simulink model "CntroInput"  (R2016b)
settings: Solver=FixedStepAuto  StartTime=0.0  StopTime=10.0  RelTol=1e-3  SampleTimeConstraint=STIndependent
undefined symbols (not defined in the file): MPCSampleTime
libraries: simulink x7
settings Model: Creator=UAVLAB  LastModifiedBy=UAVLAB

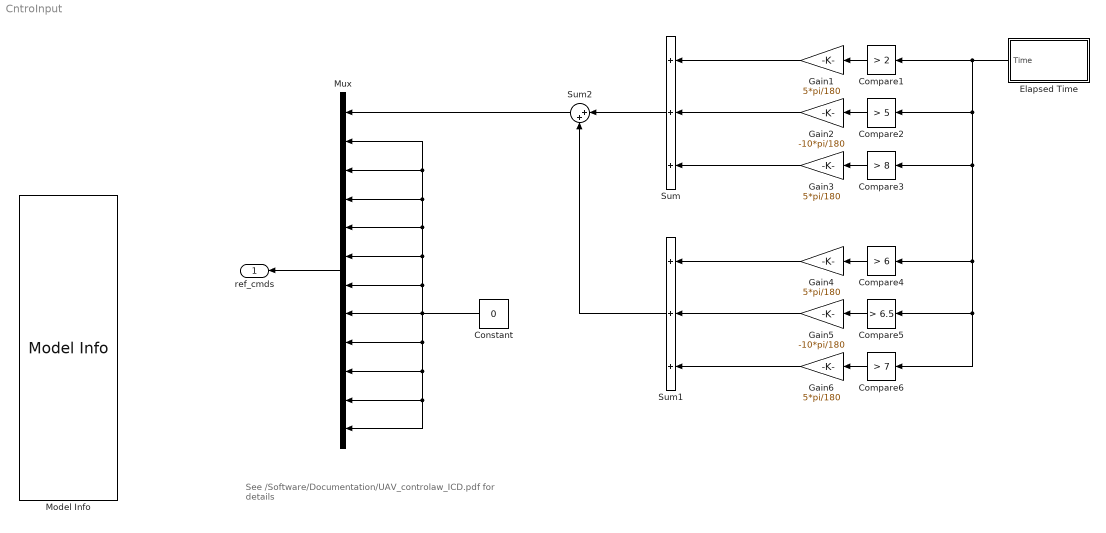
== system CntroInput ==
  note: See /Software/Documentation/UAV_controlaw_ICD.pdf
      | for details
  Compare1 : simulink/Logic and Bit Operations/Compare To Constant  relop=>  const=2  OutDataTypeStr=boolean
  Compare2 : simulink/Logic and Bit Operations/Compare To Constant  relop=>  const=5  OutDataTypeStr=boolean
  Compare3 : simulink/Logic and Bit Operations/Compare To Constant  relop=>  const=8  OutDataTypeStr=boolean
  Compare4 : simulink/Logic and Bit Operations/Compare To Constant  relop=>  const=6  OutDataTypeStr=boolean
  Compare5 : simulink/Logic and Bit Operations/Compare To Constant  relop=>  const=6.5  OutDataTypeStr=boolean
  Compare6 : simulink/Logic and Bit Operations/Compare To Constant  relop=>  const=7  OutDataTypeStr=boolean
  Constant : Constant  Value=0  SampleTime=-1
  Elapsed Time : Subsystem
  Gain{1,3..4,6} (4 alike) : Gain  Gain=5*pi/180  OutDataTypeStr=double
  Gain2 : Gain  Gain=-10*pi/180  OutDataTypeStr=double
  Gain5 : Gain  Gain=-10*pi/180  OutDataTypeStr=double
  Model Info : simulink/Model-Wide Utilities/Model Info  Frame=on  DisplayStringWithTags=|  HorizontalTextAlignment=Center  LeftAlignmentValue=0.5  SourceBlockDiagram=control_input2  TagMaxNumber=20
      | Ref Cmd Port Info
      | 
      | 1. phi_cmd
      | 2. theta_cmd
      | 3. psi_cmd
      | 4. p_cmd
      | 5. q_cmd
      | 6. r_cmd
      | 7. V_s_cmd
      | 8. h_cmd
      | 9. gndtrk_cmd
      | 10. aoa_cmd
      | 11. aos_cmd
      | 12. gamma_cmd
  Mux : Mux  Inputs=12
  Sum : Sum  Inputs=+++
  Sum1 : Sum  Inputs=+++
  Sum2 : Sum  Inputs=|++
  ref_cmds : Outport
  wires:
  Mux/1 -> ref_cmds/1
  Constant/1 -> Mux/2, Mux/3, Mux/4, Mux/5, Mux/6, Mux/7, Mux/8, Mux/9, Mux/10, Mux/11, Mux/12
  Sum/1 -> Sum2/1
  Sum2/1 -> Mux/1
  Compare1/1 -> Gain1/1
  Gain1/1 -> Sum/1
  Compare2/1 -> Gain2/1
  Gain2/1 -> Sum/2
  Compare3/1 -> Gain3/1
  Gain3/1 -> Sum/3
  Elapsed Time/1(Time) -> Compare4/1, Compare5/1, Compare6/1, Compare3/1, Compare2/1, Compare1/1
  Compare4/1 -> Gain4/1
  Gain4/1 -> Sum1/1
  Compare5/1 -> Gain5/1
  Gain5/1 -> Sum1/2
  Compare6/1 -> Gain6/1
  Gain6/1 -> Sum1/3
  Sum1/1 -> Sum2/2

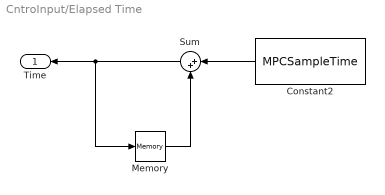
== system CntroInput/Elapsed Time ==
  Constant2 : Constant  Value=MPCSampleTime  SampleTime=-1
  Memory : Memory  InheritSampleTime=on
  Sum : Sum  Inputs=|++
  Time : Outport
  wires:
  Constant2/1 -> Sum/1
  Memory/1 -> Sum/2
  Sum/1 -> Memory/1, Time/1
